simulink model "systolicArrayFinal"  (R2021a)
settings: Solver=VariableStepAuto  StartTime=0.0  StopTime=13  RelTol=1e-3
libraries: hdlBasic x120, xbsIndex_r4 x1
(part 1 of 2)
settings Model: Creator=caval  LastModifiedBy=kv25

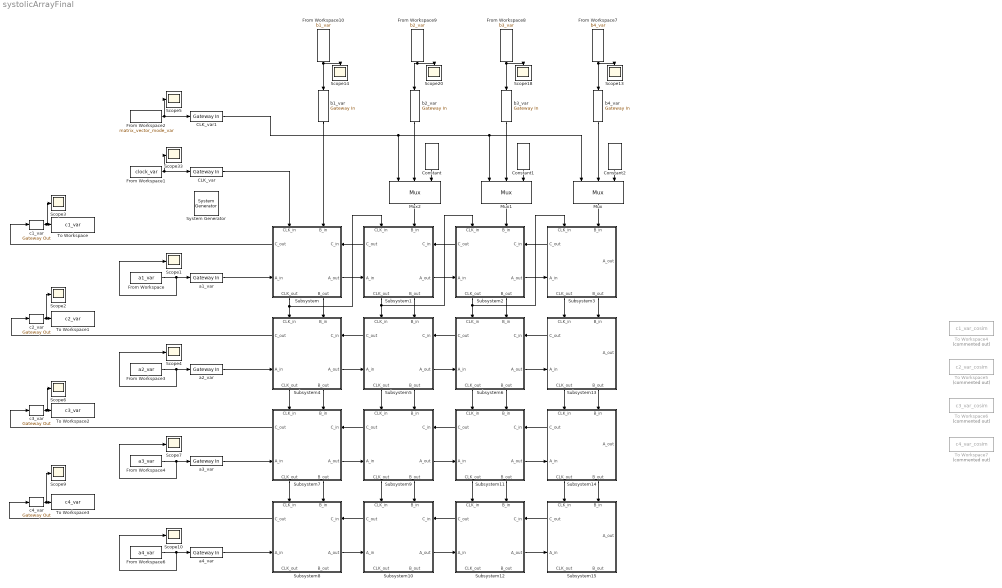
== system systolicArrayFinal ==
  " System Generator" : xbsIndex_r4/ System Generator  Tag=genX  xilinxfamily=zynq  part=xc7z020  speed=-1  package=clg484  synthesis_tool=Vivado  clock_wrapper=Clock Enables  directory=./netlist5  proj_type=Vivado  Synth_file=Vivado Synthesis Defaults  Impl_file=Vivado Implementation Defaults  testbench=off  simulink_period=1  sysclk_period=7  dcm_input_clock_period=10  incr_netlist=off  trim_vbits=Everywhere in SubSystem  dbl_ovrd=According to Block Masks  core_generation=According to Block Masks  run_coregen=off  deprecated_control=off  eval_field=0  block_type=sysgen
  CLK_var : hdlBasic/Gateway In  gui_display_data_type=Boolean  arith_type=Boolean  n_bits=16  bin_pt=0  preci_type=Single  exp_width=8  frac_width=24  rows=1  columns=1  quantization="Round  (unbiased: +/- Inf)"  overflow=Saturate  period=1  UseAsADC=off  ADCChannel='1'  interface=None  automatic_assignment=on  address_offset=hex2dec('00')  intf_name=''  intf_description=''  default_value=0  timing_constraint=None  locs_specified=off  LOCs={}  io_standard={}  inherit_from_input=off  hdl_port=on  XmcBlockStatus=1  maskContainerNames=group4  block_type=gatewayin  block_config=sysgen:gateway_in_config  block_width_w=590  block_height_w=620  block_width=640  block_height=850
  CLK_var1 : hdlBasic/Gateway In  gui_display_data_type=Boolean  arith_type=Boolean  n_bits=16  bin_pt=0  preci_type=Single  exp_width=8  frac_width=24  rows=1  columns=1  quantization="Round  (unbiased: +/- Inf)"  overflow=Saturate  period=1  UseAsADC=off  ADCChannel='1'  interface=None  automatic_assignment=on  address_offset=hex2dec('00')  intf_name=''  intf_description=''  default_value=0  timing_constraint=None  locs_specified=off  LOCs={}  io_standard={}  inherit_from_input=off  hdl_port=on  XmcBlockStatus=1  maskContainerNames=group4  block_type=gatewayin  block_config=sysgen:gateway_in_config  block_width_w=590  block_height_w=620  block_width=640  block_height=850
  Constant : hdlBasic/Constant  const=0  gui_display_data_type=Fixed-point  arith_type=Signed (2's comp)  n_bits=16  bin_pt=0  preci_type=Single  exp_width=8  frac_width=24  explicit_period=off  period=1  XmcBlockStatus=1  maskContainerNames=tabcontainer1  block_type=constant  block_config=sysgen:Constant_config
  Constant1 : hdlBasic/Constant  const=0  gui_display_data_type=Fixed-point  arith_type=Signed (2's comp)  n_bits=16  bin_pt=0  preci_type=Single  exp_width=8  frac_width=24  explicit_period=off  period=1  XmcBlockStatus=1  maskContainerNames=tabcontainer1  block_type=constant  block_config=sysgen:Constant_config
  Constant2 : hdlBasic/Constant  const=0  gui_display_data_type=Fixed-point  arith_type=Signed (2's comp)  n_bits=16  bin_pt=0  preci_type=Single  exp_width=8  frac_width=24  explicit_period=off  period=1  XmcBlockStatus=1  maskContainerNames=tabcontainer1  block_type=constant  block_config=sysgen:Constant_config
  From Workspace : FromWorkspace  VariableName=a1_var
  From Workspace1 : FromWorkspace  VariableName=clock_var
  From Workspace10 : FromWorkspace  VariableName=b1_var
  From Workspace2 : FromWorkspace  VariableName=matrix_vector_mode_var
  From Workspace3 : FromWorkspace  VariableName=a2_var
  From Workspace4 : FromWorkspace  VariableName=a3_var
  From Workspace6 : FromWorkspace  VariableName=a4_var
  From Workspace7 : FromWorkspace  VariableName=b4_var
  From Workspace8 : FromWorkspace  VariableName=b3_var
  From Workspace9 : FromWorkspace  VariableName=b2_var
  Mux : hdlBasic/Mux  inputs=2  en=off  latency=0  precision=Full  arith_type=Unsigned  n_bits=16  bin_pt=14  quantization=Truncate  overflow=Wrap  XmcBlockStatus=1  maskContainerNames=tabcontainer1  block_type=mux  block_config=sysgen:Mux_config
  Mux1 : hdlBasic/Mux  inputs=2  en=off  latency=0  precision=Full  arith_type=Unsigned  n_bits=16  bin_pt=14  quantization=Truncate  overflow=Wrap  XmcBlockStatus=1  maskContainerNames=tabcontainer1  block_type=mux  block_config=sysgen:Mux_config
  Mux2 : hdlBasic/Mux  inputs=2  en=off  latency=0  precision=Full  arith_type=Unsigned  n_bits=16  bin_pt=14  quantization=Truncate  overflow=Wrap  XmcBlockStatus=1  maskContainerNames=tabcontainer1  block_type=mux  block_config=sysgen:Mux_config
  Scope{1..7,9..10,13..14,18,20,33} (14 alike) : Scope
      Scope2 settings: Description=C14  AttributesFormatString=texttest
      Scope3 settings: Description=C14  AttributesFormatString=texttest
      Scope6 settings: Description=C14  AttributesFormatString=texttest
      Scope9 settings: Description=C14  AttributesFormatString=texttest
  Subsystem : Subsystem
      settings: PortSchema="{\"entries\":[{\"content\":{\"sides\":[{\"content\":{\"connectorIds\":[\"In1\",\"In2\"]},\"type\":\"ConnectorPlacement.EquallySpacedRectSide\",\"uuid\":\"d43d3dc0-f2a2-4485-9cc8-fdcdc63c7c64\"},{\"content\":{\"connectorIds\":[\"Out1\",\"Out2\"],\"side\":\"RIGHT\"},\"type\":\"ConnectorPlacement.EquallySpacedRectSide\",\"uuid\":\"56044226-4723-40c7-a478-8333213a0054\"},{\"content\":{\"connectorIds\":[\"Out4\",\"In3\"],\"side\":\"TOP\"},\"type\":\"ConnectorPlacement.EquallySpacedRectSide\",\"uuid\":\"fc372aae-6eb0-4644-b08a-28c78073ed8c\"},{\"content\":{\"connectorIds\":[\"In4\",\"Out3\"],\"side\":\"BOTTOM\"},\"type\":\"ConnectorPlacement.EquallySpacedRectSide\",\"uuid\":\"a99b4862-bd6b-40ce-bb78-73155b1cda06\"}]},\"type\":\"ConnectorPlacement.EquallySpacedConnector\",\"uuid\":\"00547539-55f6-42ab-bc8f-0525219f70ea\"}],\"packageUris\":[\"http://schema.mathworks.com/mf0/Connector/R2020b\"],\"version\":\"1.0\"}"
  Subsystem1 : Subsystem
      settings: PortSchema="{\"entries\":[{\"content\":{\"sides\":[{\"content\":{\"connectorIds\":[\"In1\",\"In2\"]},\"type\":\"ConnectorPlacement.EquallySpacedRectSide\",\"uuid\":\"d43d3dc0-f2a2-4485-9cc8-fdcdc63c7c64\"},{\"content\":{\"connectorIds\":[\"Out1\",\"Out2\"],\"side\":\"RIGHT\"},\"type\":\"ConnectorPlacement.EquallySpacedRectSide\",\"uuid\":\"56044226-4723-40c7-a478-8333213a0054\"},{\"content\":{\"connectorIds\":[\"Out4\",\"In3\"],\"side\":\"TOP\"},\"type\":\"ConnectorPlacement.EquallySpacedRectSide\",\"uuid\":\"fc372aae-6eb0-4644-b08a-28c78073ed8c\"},{\"content\":{\"connectorIds\":[\"In4\",\"Out3\"],\"side\":\"BOTTOM\"},\"type\":\"ConnectorPlacement.EquallySpacedRectSide\",\"uuid\":\"a99b4862-bd6b-40ce-bb78-73155b1cda06\"}]},\"type\":\"ConnectorPlacement.EquallySpacedConnector\",\"uuid\":\"00547539-55f6-42ab-bc8f-0525219f70ea\"}],\"packageUris\":[\"http://schema.mathworks.com/mf0/Connector/R2020b\"],\"version\":\"1.0\"}"
  Subsystem10 : Subsystem
      settings: PortSchema="{\"entries\":[{\"content\":{\"sides\":[{\"content\":{\"connectorIds\":[\"In1\",\"In2\"]},\"type\":\"ConnectorPlacement.EquallySpacedRectSide\",\"uuid\":\"d43d3dc0-f2a2-4485-9cc8-fdcdc63c7c64\"},{\"content\":{\"connectorIds\":[\"Out1\",\"Out2\"],\"side\":\"RIGHT\"},\"type\":\"ConnectorPlacement.EquallySpacedRectSide\",\"uuid\":\"56044226-4723-40c7-a478-8333213a0054\"},{\"content\":{\"connectorIds\":[\"Out4\",\"In3\"],\"side\":\"TOP\"},\"type\":\"ConnectorPlacement.EquallySpacedRectSide\",\"uuid\":\"fc372aae-6eb0-4644-b08a-28c78073ed8c\"},{\"content\":{\"connectorIds\":[\"In4\",\"Out3\"],\"side\":\"BOTTOM\"},\"type\":\"ConnectorPlacement.EquallySpacedRectSide\",\"uuid\":\"a99b4862-bd6b-40ce-bb78-73155b1cda06\"}]},\"type\":\"ConnectorPlacement.EquallySpacedConnector\",\"uuid\":\"00547539-55f6-42ab-bc8f-0525219f70ea\"}],\"packageUris\":[\"http://schema.mathworks.com/mf0/Connector/R2020b\"],\"version\":\"1.0\"}"
  Subsystem11 : Subsystem
      settings: PortSchema="{\"entries\":[{\"content\":{\"sides\":[{\"content\":{\"connectorIds\":[\"In1\",\"In2\"]},\"type\":\"ConnectorPlacement.EquallySpacedRectSide\",\"uuid\":\"d43d3dc0-f2a2-4485-9cc8-fdcdc63c7c64\"},{\"content\":{\"connectorIds\":[\"Out1\",\"Out2\"],\"side\":\"RIGHT\"},\"type\":\"ConnectorPlacement.EquallySpacedRectSide\",\"uuid\":\"56044226-4723-40c7-a478-8333213a0054\"},{\"content\":{\"connectorIds\":[\"Out4\",\"In3\"],\"side\":\"TOP\"},\"type\":\"ConnectorPlacement.EquallySpacedRectSide\",\"uuid\":\"fc372aae-6eb0-4644-b08a-28c78073ed8c\"},{\"content\":{\"connectorIds\":[\"In4\",\"Out3\"],\"side\":\"BOTTOM\"},\"type\":\"ConnectorPlacement.EquallySpacedRectSide\",\"uuid\":\"a99b4862-bd6b-40ce-bb78-73155b1cda06\"}]},\"type\":\"ConnectorPlacement.EquallySpacedConnector\",\"uuid\":\"00547539-55f6-42ab-bc8f-0525219f70ea\"}],\"packageUris\":[\"http://schema.mathworks.com/mf0/Connector/R2020b\"],\"version\":\"1.0\"}"
  Subsystem12 : Subsystem
      settings: PortSchema="{\"entries\":[{\"content\":{\"sides\":[{\"content\":{\"connectorIds\":[\"In1\",\"In2\"]},\"type\":\"ConnectorPlacement.EquallySpacedRectSide\",\"uuid\":\"d43d3dc0-f2a2-4485-9cc8-fdcdc63c7c64\"},{\"content\":{\"connectorIds\":[\"Out1\",\"Out2\"],\"side\":\"RIGHT\"},\"type\":\"ConnectorPlacement.EquallySpacedRectSide\",\"uuid\":\"56044226-4723-40c7-a478-8333213a0054\"},{\"content\":{\"connectorIds\":[\"Out4\",\"In3\"],\"side\":\"TOP\"},\"type\":\"ConnectorPlacement.EquallySpacedRectSide\",\"uuid\":\"fc372aae-6eb0-4644-b08a-28c78073ed8c\"},{\"content\":{\"connectorIds\":[\"In4\",\"Out3\"],\"side\":\"BOTTOM\"},\"type\":\"ConnectorPlacement.EquallySpacedRectSide\",\"uuid\":\"a99b4862-bd6b-40ce-bb78-73155b1cda06\"}]},\"type\":\"ConnectorPlacement.EquallySpacedConnector\",\"uuid\":\"00547539-55f6-42ab-bc8f-0525219f70ea\"}],\"packageUris\":[\"http://schema.mathworks.com/mf0/Connector/R2020b\"],\"version\":\"1.0\"}"
  Subsystem13 : Subsystem
      settings: PortSchema="{\"entries\":[{\"content\":{\"sides\":[{\"content\":{\"connectorIds\":[\"In1\",\"In2\"]},\"type\":\"ConnectorPlacement.EquallySpacedRectSide\",\"uuid\":\"d43d3dc0-f2a2-4485-9cc8-fdcdc63c7c64\"},{\"content\":{\"connectorIds\":[\"Out1\",\"Out2\"],\"side\":\"RIGHT\"},\"type\":\"ConnectorPlacement.EquallySpacedRectSide\",\"uuid\":\"56044226-4723-40c7-a478-8333213a0054\"},{\"content\":{\"connectorIds\":[\"Out4\",\"In3\"],\"side\":\"TOP\"},\"type\":\"ConnectorPlacement.EquallySpacedRectSide\",\"uuid\":\"fc372aae-6eb0-4644-b08a-28c78073ed8c\"},{\"content\":{\"connectorIds\":[\"Out3\"],\"side\":\"BOTTOM\"},\"type\":\"ConnectorPlacement.EquallySpacedRectSide\",\"uuid\":\"a99b4862-bd6b-40ce-bb78-73155b1cda06\"}]},\"type\":\"ConnectorPlacement.EquallySpacedConnector\",\"uuid\":\"00547539-55f6-42ab-bc8f-0525219f70ea\"}],\"packageUris\":[\"http://schema.mathworks.com/mf0/Connector/R2020b\"],\"version\":\"1.0\"}"
  Subsystem14 : Subsystem
      settings: PortSchema="{\"entries\":[{\"content\":{\"sides\":[{\"content\":{\"connectorIds\":[\"In1\",\"In2\"]},\"type\":\"ConnectorPlacement.EquallySpacedRectSide\",\"uuid\":\"d43d3dc0-f2a2-4485-9cc8-fdcdc63c7c64\"},{\"content\":{\"connectorIds\":[\"Out1\",\"Out2\"],\"side\":\"RIGHT\"},\"type\":\"ConnectorPlacement.EquallySpacedRectSide\",\"uuid\":\"56044226-4723-40c7-a478-8333213a0054\"},{\"content\":{\"connectorIds\":[\"Out4\",\"In3\"],\"side\":\"TOP\"},\"type\":\"ConnectorPlacement.EquallySpacedRectSide\",\"uuid\":\"fc372aae-6eb0-4644-b08a-28c78073ed8c\"},{\"content\":{\"connectorIds\":[\"Out3\"],\"side\":\"BOTTOM\"},\"type\":\"ConnectorPlacement.EquallySpacedRectSide\",\"uuid\":\"a99b4862-bd6b-40ce-bb78-73155b1cda06\"}]},\"type\":\"ConnectorPlacement.EquallySpacedConnector\",\"uuid\":\"00547539-55f6-42ab-bc8f-0525219f70ea\"}],\"packageUris\":[\"http://schema.mathworks.com/mf0/Connector/R2020b\"],\"version\":\"1.0\"}"
  Subsystem15 : Subsystem
      settings: PortSchema="{\"entries\":[{\"content\":{\"sides\":[{\"content\":{\"connectorIds\":[\"In1\",\"In2\"]},\"type\":\"ConnectorPlacement.EquallySpacedRectSide\",\"uuid\":\"d43d3dc0-f2a2-4485-9cc8-fdcdc63c7c64\"},{\"content\":{\"connectorIds\":[\"Out1\",\"Out2\"],\"side\":\"RIGHT\"},\"type\":\"ConnectorPlacement.EquallySpacedRectSide\",\"uuid\":\"56044226-4723-40c7-a478-8333213a0054\"},{\"content\":{\"connectorIds\":[\"Out4\",\"In3\"],\"side\":\"TOP\"},\"type\":\"ConnectorPlacement.EquallySpacedRectSide\",\"uuid\":\"fc372aae-6eb0-4644-b08a-28c78073ed8c\"},{\"content\":{\"connectorIds\":[\"Out3\"],\"side\":\"BOTTOM\"},\"type\":\"ConnectorPlacement.EquallySpacedRectSide\",\"uuid\":\"a99b4862-bd6b-40ce-bb78-73155b1cda06\"}]},\"type\":\"ConnectorPlacement.EquallySpacedConnector\",\"uuid\":\"00547539-55f6-42ab-bc8f-0525219f70ea\"}],\"packageUris\":[\"http://schema.mathworks.com/mf0/Connector/R2020b\"],\"version\":\"1.0\"}"
  Subsystem2 : Subsystem
      settings: PortSchema="{\"entries\":[{\"content\":{\"sides\":[{\"content\":{\"connectorIds\":[\"In1\",\"In2\"]},\"type\":\"ConnectorPlacement.EquallySpacedRectSide\",\"uuid\":\"d43d3dc0-f2a2-4485-9cc8-fdcdc63c7c64\"},{\"content\":{\"connectorIds\":[\"Out1\",\"Out2\"],\"side\":\"RIGHT\"},\"type\":\"ConnectorPlacement.EquallySpacedRectSide\",\"uuid\":\"56044226-4723-40c7-a478-8333213a0054\"},{\"content\":{\"connectorIds\":[\"Out4\",\"In3\"],\"side\":\"TOP\"},\"type\":\"ConnectorPlacement.EquallySpacedRectSide\",\"uuid\":\"fc372aae-6eb0-4644-b08a-28c78073ed8c\"},{\"content\":{\"connectorIds\":[\"In4\",\"Out3\"],\"side\":\"BOTTOM\"},\"type\":\"ConnectorPlacement.EquallySpacedRectSide\",\"uuid\":\"a99b4862-bd6b-40ce-bb78-73155b1cda06\"}]},\"type\":\"ConnectorPlacement.EquallySpacedConnector\",\"uuid\":\"00547539-55f6-42ab-bc8f-0525219f70ea\"}],\"packageUris\":[\"http://schema.mathworks.com/mf0/Connector/R2020b\"],\"version\":\"1.0\"}"
  Subsystem3 : Subsystem
      settings: PortSchema="{\"entries\":[{\"content\":{\"sides\":[{\"content\":{\"connectorIds\":[\"In1\",\"In2\"]},\"type\":\"ConnectorPlacement.EquallySpacedRectSide\",\"uuid\":\"d43d3dc0-f2a2-4485-9cc8-fdcdc63c7c64\"},{\"content\":{\"connectorIds\":[\"Out1\",\"Out2\"],\"side\":\"RIGHT\"},\"type\":\"ConnectorPlacement.EquallySpacedRectSide\",\"uuid\":\"56044226-4723-40c7-a478-8333213a0054\"},{\"content\":{\"connectorIds\":[\"Out4\",\"In3\"],\"side\":\"TOP\"},\"type\":\"ConnectorPlacement.EquallySpacedRectSide\",\"uuid\":\"fc372aae-6eb0-4644-b08a-28c78073ed8c\"},{\"content\":{\"connectorIds\":[\"Out3\"],\"side\":\"BOTTOM\"},\"type\":\"ConnectorPlacement.EquallySpacedRectSide\",\"uuid\":\"a99b4862-bd6b-40ce-bb78-73155b1cda06\"}]},\"type\":\"ConnectorPlacement.EquallySpacedConnector\",\"uuid\":\"00547539-55f6-42ab-bc8f-0525219f70ea\"}],\"packageUris\":[\"http://schema.mathworks.com/mf0/Connector/R2020b\"],\"version\":\"1.0\"}"
  Subsystem4 : Subsystem
      settings: PortSchema="{\"entries\":[{\"content\":{\"sides\":[{\"content\":{\"connectorIds\":[\"In1\",\"In2\"]},\"type\":\"ConnectorPlacement.EquallySpacedRectSide\",\"uuid\":\"d43d3dc0-f2a2-4485-9cc8-fdcdc63c7c64\"},{\"content\":{\"connectorIds\":[\"Out1\",\"Out2\"],\"side\":\"RIGHT\"},\"type\":\"ConnectorPlacement.EquallySpacedRectSide\",\"uuid\":\"56044226-4723-40c7-a478-8333213a0054\"},{\"content\":{\"connectorIds\":[\"Out4\",\"In3\"],\"side\":\"TOP\"},\"type\":\"ConnectorPlacement.EquallySpacedRectSide\",\"uuid\":\"fc372aae-6eb0-4644-b08a-28c78073ed8c\"},{\"content\":{\"connectorIds\":[\"In4\",\"Out3\"],\"side\":\"BOTTOM\"},\"type\":\"ConnectorPlacement.EquallySpacedRectSide\",\"uuid\":\"a99b4862-bd6b-40ce-bb78-73155b1cda06\"}]},\"type\":\"ConnectorPlacement.EquallySpacedConnector\",\"uuid\":\"00547539-55f6-42ab-bc8f-0525219f70ea\"}],\"packageUris\":[\"http://schema.mathworks.com/mf0/Connector/R2020b\"],\"version\":\"1.0\"}"
  Subsystem5 : Subsystem
      settings: PortSchema="{\"entries\":[{\"content\":{\"sides\":[{\"content\":{\"connectorIds\":[\"In1\",\"In2\"]},\"type\":\"ConnectorPlacement.EquallySpacedRectSide\",\"uuid\":\"d43d3dc0-f2a2-4485-9cc8-fdcdc63c7c64\"},{\"content\":{\"connectorIds\":[\"Out1\",\"Out2\"],\"side\":\"RIGHT\"},\"type\":\"ConnectorPlacement.EquallySpacedRectSide\",\"uuid\":\"56044226-4723-40c7-a478-8333213a0054\"},{\"content\":{\"connectorIds\":[\"Out4\",\"In3\"],\"side\":\"TOP\"},\"type\":\"ConnectorPlacement.EquallySpacedRectSide\",\"uuid\":\"fc372aae-6eb0-4644-b08a-28c78073ed8c\"},{\"content\":{\"connectorIds\":[\"In4\",\"Out3\"],\"side\":\"BOTTOM\"},\"type\":\"ConnectorPlacement.EquallySpacedRectSide\",\"uuid\":\"a99b4862-bd6b-40ce-bb78-73155b1cda06\"}]},\"type\":\"ConnectorPlacement.EquallySpacedConnector\",\"uuid\":\"00547539-55f6-42ab-bc8f-0525219f70ea\"}],\"packageUris\":[\"http://schema.mathworks.com/mf0/Connector/R2020b\"],\"version\":\"1.0\"}"
  Subsystem6 : Subsystem
      settings: PortSchema="{\"entries\":[{\"content\":{\"sides\":[{\"content\":{\"connectorIds\":[\"In1\",\"In2\"]},\"type\":\"ConnectorPlacement.EquallySpacedRectSide\",\"uuid\":\"d43d3dc0-f2a2-4485-9cc8-fdcdc63c7c64\"},{\"content\":{\"connectorIds\":[\"Out1\",\"Out2\"],\"side\":\"RIGHT\"},\"type\":\"ConnectorPlacement.EquallySpacedRectSide\",\"uuid\":\"56044226-4723-40c7-a478-8333213a0054\"},{\"content\":{\"connectorIds\":[\"Out4\",\"In3\"],\"side\":\"TOP\"},\"type\":\"ConnectorPlacement.EquallySpacedRectSide\",\"uuid\":\"fc372aae-6eb0-4644-b08a-28c78073ed8c\"},{\"content\":{\"connectorIds\":[\"In4\",\"Out3\"],\"side\":\"BOTTOM\"},\"type\":\"ConnectorPlacement.EquallySpacedRectSide\",\"uuid\":\"a99b4862-bd6b-40ce-bb78-73155b1cda06\"}]},\"type\":\"ConnectorPlacement.EquallySpacedConnector\",\"uuid\":\"00547539-55f6-42ab-bc8f-0525219f70ea\"}],\"packageUris\":[\"http://schema.mathworks.com/mf0/Connector/R2020b\"],\"version\":\"1.0\"}"
  Subsystem7 : Subsystem
      settings: PortSchema="{\"entries\":[{\"content\":{\"sides\":[{\"content\":{\"connectorIds\":[\"In1\",\"In2\"]},\"type\":\"ConnectorPlacement.EquallySpacedRectSide\",\"uuid\":\"d43d3dc0-f2a2-4485-9cc8-fdcdc63c7c64\"},{\"content\":{\"connectorIds\":[\"Out1\",\"Out2\"],\"side\":\"RIGHT\"},\"type\":\"ConnectorPlacement.EquallySpacedRectSide\",\"uuid\":\"56044226-4723-40c7-a478-8333213a0054\"},{\"content\":{\"connectorIds\":[\"Out4\",\"In3\"],\"side\":\"TOP\"},\"type\":\"ConnectorPlacement.EquallySpacedRectSide\",\"uuid\":\"fc372aae-6eb0-4644-b08a-28c78073ed8c\"},{\"content\":{\"connectorIds\":[\"In4\",\"Out3\"],\"side\":\"BOTTOM\"},\"type\":\"ConnectorPlacement.EquallySpacedRectSide\",\"uuid\":\"a99b4862-bd6b-40ce-bb78-73155b1cda06\"}]},\"type\":\"ConnectorPlacement.EquallySpacedConnector\",\"uuid\":\"00547539-55f6-42ab-bc8f-0525219f70ea\"}],\"packageUris\":[\"http://schema.mathworks.com/mf0/Connector/R2020b\"],\"version\":\"1.0\"}"
  Subsystem8 : Subsystem
      settings: PortSchema="{\"entries\":[{\"content\":{\"sides\":[{\"content\":{\"connectorIds\":[\"In1\",\"In2\"]},\"type\":\"ConnectorPlacement.EquallySpacedRectSide\",\"uuid\":\"d43d3dc0-f2a2-4485-9cc8-fdcdc63c7c64\"},{\"content\":{\"connectorIds\":[\"Out1\",\"Out2\"],\"side\":\"RIGHT\"},\"type\":\"ConnectorPlacement.EquallySpacedRectSide\",\"uuid\":\"56044226-4723-40c7-a478-8333213a0054\"},{\"content\":{\"connectorIds\":[\"Out4\",\"In3\"],\"side\":\"TOP\"},\"type\":\"ConnectorPlacement.EquallySpacedRectSide\",\"uuid\":\"fc372aae-6eb0-4644-b08a-28c78073ed8c\"},{\"content\":{\"connectorIds\":[\"In4\",\"Out3\"],\"side\":\"BOTTOM\"},\"type\":\"ConnectorPlacement.EquallySpacedRectSide\",\"uuid\":\"a99b4862-bd6b-40ce-bb78-73155b1cda06\"}]},\"type\":\"ConnectorPlacement.EquallySpacedConnector\",\"uuid\":\"00547539-55f6-42ab-bc8f-0525219f70ea\"}],\"packageUris\":[\"http://schema.mathworks.com/mf0/Connector/R2020b\"],\"version\":\"1.0\"}"
  Subsystem9 : Subsystem
      settings: PortSchema="{\"entries\":[{\"content\":{\"sides\":[{\"content\":{\"connectorIds\":[\"In1\",\"In2\"]},\"type\":\"ConnectorPlacement.EquallySpacedRectSide\",\"uuid\":\"d43d3dc0-f2a2-4485-9cc8-fdcdc63c7c64\"},{\"content\":{\"connectorIds\":[\"Out1\",\"Out2\"],\"side\":\"RIGHT\"},\"type\":\"ConnectorPlacement.EquallySpacedRectSide\",\"uuid\":\"56044226-4723-40c7-a478-8333213a0054\"},{\"content\":{\"connectorIds\":[\"Out4\",\"In3\"],\"side\":\"TOP\"},\"type\":\"ConnectorPlacement.EquallySpacedRectSide\",\"uuid\":\"fc372aae-6eb0-4644-b08a-28c78073ed8c\"},{\"content\":{\"connectorIds\":[\"In4\",\"Out3\"],\"side\":\"BOTTOM\"},\"type\":\"ConnectorPlacement.EquallySpacedRectSide\",\"uuid\":\"a99b4862-bd6b-40ce-bb78-73155b1cda06\"}]},\"type\":\"ConnectorPlacement.EquallySpacedConnector\",\"uuid\":\"00547539-55f6-42ab-bc8f-0525219f70ea\"}],\"packageUris\":[\"http://schema.mathworks.com/mf0/Connector/R2020b\"],\"version\":\"1.0\"}"
  To Workspace : ToWorkspace  VariableName=c1_var  SaveFormat=Timeseries  SampleTime=-1
  To Workspace1 : ToWorkspace  VariableName=c2_var  SaveFormat=Timeseries  SampleTime=-1
  To Workspace2 : ToWorkspace  VariableName=c3_var  SaveFormat=Timeseries  SampleTime=-1
  To Workspace3 : ToWorkspace  VariableName=c4_var  SaveFormat=Timeseries  SampleTime=-1
  To Workspace4 : ToWorkspace  Commented=on  VariableName=c1_var_cosim  SaveFormat=Timeseries  SampleTime=-1
  To Workspace5 : ToWorkspace  Commented=on  VariableName=c2_var_cosim  SaveFormat=Timeseries  SampleTime=-1
  To Workspace6 : ToWorkspace  Commented=on  VariableName=c3_var_cosim  SaveFormat=Timeseries  SampleTime=-1
  To Workspace7 : ToWorkspace  Commented=on  VariableName=c4_var_cosim  SaveFormat=Timeseries  SampleTime=-1
  a1_var : hdlBasic/Gateway In  gui_display_data_type=Fixed-point  arith_type=Signed (2's comp)  n_bits=16  bin_pt=0  preci_type=Single  exp_width=8  frac_width=24  rows=1  columns=1  quantization="Round  (unbiased: +/- Inf)"  overflow=Saturate  period=1  UseAsADC=off  ADCChannel='1'  interface=None  automatic_assignment=on  address_offset=hex2dec('00')  intf_name=''  intf_description=''  default_value=0  timing_constraint=None  locs_specified=off  LOCs={}  io_standard={}  inherit_from_input=off  hdl_port=on  XmcBlockStatus=1  maskContainerNames=group4  block_type=gatewayin  block_config=sysgen:gateway_in_config  block_width_w=590  block_height_w=620  block_width=640  block_height=850
  a2_var : hdlBasic/Gateway In  gui_display_data_type=Fixed-point  arith_type=Signed (2's comp)  n_bits=16  bin_pt=0  preci_type=Single  exp_width=8  frac_width=24  rows=1  columns=1  quantization="Round  (unbiased: +/- Inf)"  overflow=Saturate  period=1  UseAsADC=off  ADCChannel='1'  interface=None  automatic_assignment=on  address_offset=hex2dec('00')  intf_name=''  intf_description=''  default_value=0  timing_constraint=None  locs_specified=off  LOCs={}  io_standard={}  inherit_from_input=off  hdl_port=on  XmcBlockStatus=1  maskContainerNames=group4  block_type=gatewayin  block_config=sysgen:gateway_in_config  block_width_w=590  block_height_w=620  block_width=640  block_height=850
  a3_var : hdlBasic/Gateway In  gui_display_data_type=Fixed-point  arith_type=Signed (2's comp)  n_bits=16  bin_pt=0  preci_type=Single  exp_width=8  frac_width=24  rows=1  columns=1  quantization="Round  (unbiased: +/- Inf)"  overflow=Saturate  period=1  UseAsADC=off  ADCChannel='1'  interface=None  automatic_assignment=on  address_offset=hex2dec('00')  intf_name=''  intf_description=''  default_value=0  timing_constraint=None  locs_specified=off  LOCs={}  io_standard={}  inherit_from_input=off  hdl_port=on  XmcBlockStatus=1  maskContainerNames=group4  block_type=gatewayin  block_config=sysgen:gateway_in_config  block_width_w=590  block_height_w=620  block_width=640  block_height=850
  a4_var : hdlBasic/Gateway In  gui_display_data_type=Fixed-point  arith_type=Signed (2's comp)  n_bits=16  bin_pt=0  preci_type=Single  exp_width=8  frac_width=24  rows=1  columns=1  quantization="Round  (unbiased: +/- Inf)"  overflow=Saturate  period=1  UseAsADC=off  ADCChannel='1'  interface=None  automatic_assignment=on  address_offset=hex2dec('00')  intf_name=''  intf_description=''  default_value=0  timing_constraint=None  locs_specified=off  LOCs={}  io_standard={}  inherit_from_input=off  hdl_port=on  XmcBlockStatus=1  maskContainerNames=group4  block_type=gatewayin  block_config=sysgen:gateway_in_config  block_width_w=590  block_height_w=620  block_width=640  block_height=850
  b1_var : hdlBasic/Gateway In  gui_display_data_type=Fixed-point  arith_type=Signed (2's comp)  n_bits=16  bin_pt=0  preci_type=Single  exp_width=8  frac_width=24  rows=1  columns=1  quantization="Round  (unbiased: +/- Inf)"  overflow=Saturate  period=1  UseAsADC=off  ADCChannel='1'  interface=None  automatic_assignment=on  address_offset=hex2dec('00')  intf_name=''  intf_description=''  default_value=0  timing_constraint=None  locs_specified=off  LOCs={}  io_standard={}  inherit_from_input=off  hdl_port=on  XmcBlockStatus=1  maskContainerNames=group4  block_type=gatewayin  block_config=sysgen:gateway_in_config  block_width_w=590  block_height_w=620  block_width=640  block_height=850
  b2_var : hdlBasic/Gateway In  gui_display_data_type=Fixed-point  arith_type=Signed (2's comp)  n_bits=16  bin_pt=0  preci_type=Single  exp_width=8  frac_width=24  rows=1  columns=1  quantization="Round  (unbiased: +/- Inf)"  overflow=Saturate  period=1  UseAsADC=off  ADCChannel='1'  interface=None  automatic_assignment=on  address_offset=hex2dec('00')  intf_name=''  intf_description=''  default_value=0  timing_constraint=None  locs_specified=off  LOCs={}  io_standard={}  inherit_from_input=off  hdl_port=on  XmcBlockStatus=1  maskContainerNames=group4  block_type=gatewayin  block_config=sysgen:gateway_in_config  block_width_w=590  block_height_w=620  block_width=640  block_height=850
  b3_var : hdlBasic/Gateway In  gui_display_data_type=Fixed-point  arith_type=Signed (2's comp)  n_bits=16  bin_pt=0  preci_type=Single  exp_width=8  frac_width=24  rows=1  columns=1  quantization="Round  (unbiased: +/- Inf)"  overflow=Saturate  period=1  UseAsADC=off  ADCChannel='1'  interface=None  automatic_assignment=on  address_offset=hex2dec('00')  intf_name=''  intf_description=''  default_value=0  timing_constraint=None  locs_specified=off  LOCs={}  io_standard={}  inherit_from_input=off  hdl_port=on  XmcBlockStatus=1  maskContainerNames=group4  block_type=gatewayin  block_config=sysgen:gateway_in_config  block_width_w=590  block_height_w=620  block_width=640  block_height=850
  b4_var : hdlBasic/Gateway In  gui_display_data_type=Fixed-point  arith_type=Signed (2's comp)  n_bits=16  bin_pt=0  preci_type=Single  exp_width=8  frac_width=24  rows=1  columns=1  quantization="Round  (unbiased: +/- Inf)"  overflow=Saturate  period=1  UseAsADC=off  ADCChannel='1'  interface=None  automatic_assignment=on  address_offset=hex2dec('00')  intf_name=''  intf_description=''  default_value=0  timing_constraint=None  locs_specified=off  LOCs={}  io_standard={}  inherit_from_input=off  hdl_port=on  XmcBlockStatus=1  maskContainerNames=group4  block_type=gatewayin  block_config=sysgen:gateway_in_config  block_width_w=590  block_height_w=620  block_width=640  block_height=850
  c1_var : hdlBasic/Gateway Out  inherit_from_input=off  hdl_port=on  rows=1  columns=1  UseAsDAC=off  DACChannel='1'  interface=None  automatic_assignment=on  address_offset=hex2dec('00')  intf_name=''  intf_description=''  timing_constraint=None  locs_specified=off  LOCs={}  io_standard={}  XmcBlockStatus=1  maskContainerNames=group4  block_type=gatewayout  block_config=sysgen:gateway_out_config  block_width_w=590  block_height_w=620  block_width=620  block_height=750
  c2_var : hdlBasic/Gateway Out  inherit_from_input=off  hdl_port=on  rows=1  columns=1  UseAsDAC=off  DACChannel='1'  interface=None  automatic_assignment=on  address_offset=hex2dec('00')  intf_name=''  intf_description=''  timing_constraint=None  locs_specified=off  LOCs={}  io_standard={}  XmcBlockStatus=1  maskContainerNames=group4  block_type=gatewayout  block_config=sysgen:gateway_out_config  block_width_w=590  block_height_w=620  block_width=620  block_height=750
  c3_var : hdlBasic/Gateway Out  inherit_from_input=off  hdl_port=on  rows=1  columns=1  UseAsDAC=off  DACChannel='1'  interface=None  automatic_assignment=on  address_offset=hex2dec('00')  intf_name=''  intf_description=''  timing_constraint=None  locs_specified=off  LOCs={}  io_standard={}  XmcBlockStatus=1  maskContainerNames=group4  block_type=gatewayout  block_config=sysgen:gateway_out_config  block_width_w=590  block_height_w=620  block_width=620  block_height=750
  c4_var : hdlBasic/Gateway Out  inherit_from_input=off  hdl_port=on  rows=1  columns=1  UseAsDAC=off  DACChannel='1'  interface=None  automatic_assignment=on  address_offset=hex2dec('00')  intf_name=''  intf_description=''  timing_constraint=None  locs_specified=off  LOCs={}  io_standard={}  XmcBlockStatus=1  maskContainerNames=group4  block_type=gatewayout  block_config=sysgen:gateway_out_config  block_width_w=590  block_height_w=620  block_width=620  block_height=750
  wires:
  From Workspace/1 -> Scope1/1, a1_var/1
  From Workspace3/1 -> Scope4/1, a2_var/1
  From Workspace6/1 -> Scope10/1, a4_var/1
  From Workspace4/1 -> Scope7/1, a3_var/1
  From Workspace8/1 -> Scope18/1, b3_var/1
  From Workspace10/1 -> Scope14/1, b1_var/1
  From Workspace9/1 -> Scope20/1, b2_var/1
  From Workspace7/1 -> Scope13/1, b4_var/1
  a1_var/1 -> Subsystem/3(A_in)
  Subsystem/3(A_out) -> Subsystem1/3(A_in)
  Subsystem1/3(A_out) -> Subsystem2/3(A_in)
  Subsystem2/3(A_out) -> Subsystem3/3(A_in)
  Subsystem4/3(A_out) -> Subsystem5/3(A_in)
  Subsystem5/3(A_out) -> Subsystem6/3(A_in)
  Subsystem6/3(A_out) -> Subsystem13/3(A_in)
  Subsystem7/3(A_out) -> Subsystem9/3(A_in)
  Subsystem9/3(A_out) -> Subsystem11/3(A_in)
  Subsystem11/3(A_out) -> Subsystem14/3(A_in)
  Subsystem8/3(A_out) -> Subsystem10/3(A_in)
  Subsystem10/3(A_out) -> Subsystem12/3(A_in)
  Subsystem12/3(A_out) -> Subsystem15/3(A_in)
  a2_var/1 -> Subsystem4/3(A_in)
  a3_var/1 -> Subsystem7/3(A_in)
  a4_var/1 -> Subsystem8/3(A_in)
  b1_var/1 -> Subsystem/2(B_in)
  CLK_var/1 -> Subsystem/1(CLK_in)
  Subsystem4/1(CLK_out) -> Subsystem7/1(CLK_in)
  Subsystem7/1(CLK_out) -> Subsystem8/1(CLK_in)
  Subsystem5/1(CLK_out) -> Subsystem9/1(CLK_in)
  Subsystem9/1(CLK_out) -> Subsystem10/1(CLK_in)
  Subsystem6/1(CLK_out) -> Subsystem11/1(CLK_in)
  Subsystem11/1(CLK_out) -> Subsystem12/1(CLK_in)
  Subsystem14/1(CLK_out) -> Subsystem15/1(CLK_in)
  Subsystem3/1(CLK_out) -> Subsystem13/1(CLK_in)
  Subsystem3/4(C_out) -> Subsystem2/4(C_in)
  Subsystem2/4(C_out) -> Subsystem1/4(C_in)
  Subsystem1/4(C_out) -> Subsystem/4(C_in)
  Subsystem5/4(C_out) -> Subsystem4/4(C_in)
  Subsystem6/4(C_out) -> Subsystem5/4(C_in)
  Subsystem13/4(C_out) -> Subsystem6/4(C_in)
  Subsystem9/4(C_out) -> Subsystem7/4(C_in)
  Subsystem11/4(C_out) -> Subsystem9/4(C_in)
  Subsystem14/4(C_out) -> Subsystem11/4(C_in)
  Subsystem15/4(C_out) -> Subsystem12/4(C_in)
  Subsystem12/4(C_out) -> Subsystem10/4(C_in)
  Subsystem10/4(C_out) -> Subsystem8/4(C_in)
  Subsystem8/4(C_out) -> c4_var/1
  c4_var/1 -> Scope9/1, To Workspace3/1
  c3_var/1 -> Scope6/1, To Workspace2/1
  c1_var/1 -> Scope3/1, To Workspace/1
  c2_var/1 -> Scope2/1, To Workspace1/1
  Subsystem7/4(C_out) -> c3_var/1
  Subsystem4/4(C_out) -> c2_var/1
  Subsystem/4(C_out) -> c1_var/1
  Subsystem1/2(B_out) -> Subsystem5/2(B_in)
  Subsystem5/2(B_out) -> Subsystem9/2(B_in)
  Subsystem9/2(B_out) -> Subsystem10/2(B_in)
  Subsystem11/2(B_out) -> Subsystem12/2(B_in)
  Subsystem14/2(B_out) -> Subsystem15/2(B_in)
  Subsystem6/2(B_out) -> Subsystem11/2(B_in)
  Subsystem3/2(B_out) -> Subsystem13/2(B_in)
  Subsystem2/2(B_out) -> Subsystem6/2(B_in)
  Subsystem/2(B_out) -> Subsystem4/2(B_in)
  Subsystem4/2(B_out) -> Subsystem7/2(B_in)
  Subsystem7/2(B_out) -> Subsystem8/2(B_in)
  Subsystem13/1(CLK_out) -> Subsystem14/1(CLK_in)
  Subsystem13/2(B_out) -> Subsystem14/2(B_in)
  Subsystem2/1(CLK_out) -> Subsystem3/1(CLK_in), Subsystem6/1(CLK_in)
  Subsystem1/1(CLK_out) -> Subsystem2/1(CLK_in), Subsystem5/1(CLK_in)
  Subsystem/1(CLK_out) -> Subsystem1/1(CLK_in), Subsystem4/1(CLK_in)
  From Workspace1/1 -> Scope33/1, CLK_var/1
  From Workspace2/1 -> Scope5/1, CLK_var1/1
  Mux2/1 -> Subsystem1/2(B_in)
  Mux1/1 -> Subsystem2/2(B_in)
  Mux/1 -> Subsystem3/2(B_in)
  Constant/1 -> Mux2/3
  Constant2/1 -> Mux/3
  Constant1/1 -> Mux1/3
  b2_var/1 -> Mux2/2
  b3_var/1 -> Mux1/2
  b4_var/1 -> Mux/2
  CLK_var1/1 -> Mux2/1, Mux/1, Mux1/1
  ? -> To Workspace4/1
  ? -> To Workspace5/1
  ? -> To Workspace6/1
  ? -> To Workspace7/1

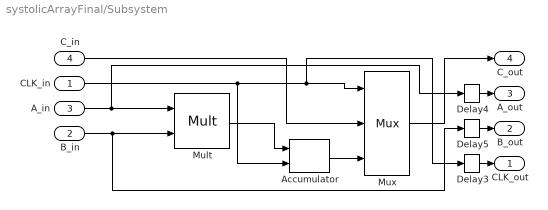
== system systolicArrayFinal/Subsystem ==
  CLK_in : Inport
  B_in : Inport  Port=2
  A_in : Inport  Port=3
  C_in : Inport  Port=4
  Accumulator : hdlBasic/Accumulator  operation=Add  n_bits=8  overflow=Wrap  scale=1  rst=on  hasbypass=off  en=off  latency=1  msb_inp=100  msb=100  lsb=-100  use_behavioral_HDL=on  implementation=Fabric  XmcBlockStatus=1  maskContainerNames=group3  block_type=accum  block_config=sysgen:Accum_config
  Delay3 : hdlBasic/Delay  rst=off  en=off  latency=1  reg_retiming=off  XmcBlockStatus=1  maskContainerNames=group1  block_type=delay  block_config=sysgen:Delay_config
  Delay4 : hdlBasic/Delay  rst=off  en=off  latency=1  reg_retiming=off  XmcBlockStatus=1  maskContainerNames=group1  block_type=delay  block_config=sysgen:Delay_config
  Delay5 : hdlBasic/Delay  rst=off  en=off  latency=1  reg_retiming=off  XmcBlockStatus=1  maskContainerNames=group1  block_type=delay  block_config=sysgen:Delay_config
  Mult : hdlBasic/Mult  precision=Full  arith_type="Signed  (2's comp)"  n_bits=16  bin_pt=14  quantization=Truncate  overflow=Wrap  en=off  latency=0  use_behavioral_HDL=off  opt=Speed  use_embedded=on  optimum_pipeline=off  pipeline=on  use_rpm=on  placement_style=Triangular  XmcBlockStatus=1  maskContainerNames=group1  block_type=mult  block_config=sysgen:Mult_config
  Mux : hdlBasic/Mux  inputs=2  en=off  latency=0  precision=Full  arith_type=Unsigned  n_bits=16  bin_pt=14  quantization=Truncate  overflow=Wrap  XmcBlockStatus=1  maskContainerNames=tabcontainer1  block_type=mux  block_config=sysgen:Mux_config
  CLK_out : Outport
  B_out : Outport  Port=2
  A_out : Outport  Port=3
  C_out : Outport  Port=4
  wires:
  Accumulator/1 -> Mux/3
  Mult/1 -> Accumulator/1
  Mux/1 -> C_out/1
  CLK_in/1 -> Accumulator/2, Delay3/1, Mux/1
  C_in/1 -> Mux/2
  A_in/1 -> Delay4/1, Mult/1
  B_in/1 -> Delay5/1, Mult/2
  Delay3/1 -> CLK_out/1
  Delay4/1 -> A_out/1
  Delay5/1 -> B_out/1

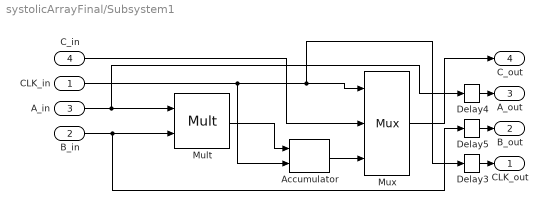
== system systolicArrayFinal/Subsystem1 ==
  CLK_in : Inport
  B_in : Inport  Port=2
  A_in : Inport  Port=3
  C_in : Inport  Port=4
  Accumulator : hdlBasic/Accumulator  operation=Add  n_bits=8  overflow=Wrap  scale=1  rst=on  hasbypass=off  en=off  latency=1  msb_inp=100  msb=100  lsb=-100  use_behavioral_HDL=on  implementation=Fabric  XmcBlockStatus=1  maskContainerNames=group3  block_type=accum  block_config=sysgen:Accum_config
  Delay3 : hdlBasic/Delay  rst=off  en=off  latency=1  reg_retiming=off  XmcBlockStatus=1  maskContainerNames=group1  block_type=delay  block_config=sysgen:Delay_config
  Delay4 : hdlBasic/Delay  rst=off  en=off  latency=1  reg_retiming=off  XmcBlockStatus=1  maskContainerNames=group1  block_type=delay  block_config=sysgen:Delay_config
  Delay5 : hdlBasic/Delay  rst=off  en=off  latency=1  reg_retiming=off  XmcBlockStatus=1  maskContainerNames=group1  block_type=delay  block_config=sysgen:Delay_config
  Mult : hdlBasic/Mult  precision=Full  arith_type="Signed  (2's comp)"  n_bits=16  bin_pt=14  quantization=Truncate  overflow=Wrap  en=off  latency=0  use_behavioral_HDL=off  opt=Speed  use_embedded=on  optimum_pipeline=off  pipeline=on  use_rpm=on  placement_style=Triangular  XmcBlockStatus=1  maskContainerNames=group1  block_type=mult  block_config=sysgen:Mult_config
  Mux : hdlBasic/Mux  inputs=2  en=off  latency=0  precision=Full  arith_type=Unsigned  n_bits=16  bin_pt=14  quantization=Truncate  overflow=Wrap  XmcBlockStatus=1  maskContainerNames=tabcontainer1  block_type=mux  block_config=sysgen:Mux_config
  CLK_out : Outport
  B_out : Outport  Port=2
  A_out : Outport  Port=3
  C_out : Outport  Port=4
  wires:
  Accumulator/1 -> Mux/3
  Mult/1 -> Accumulator/1
  Mux/1 -> C_out/1
  CLK_in/1 -> Accumulator/2, Delay3/1, Mux/1
  C_in/1 -> Mux/2
  A_in/1 -> Delay4/1, Mult/1
  B_in/1 -> Delay5/1, Mult/2
  Delay3/1 -> CLK_out/1
  Delay4/1 -> A_out/1
  Delay5/1 -> B_out/1

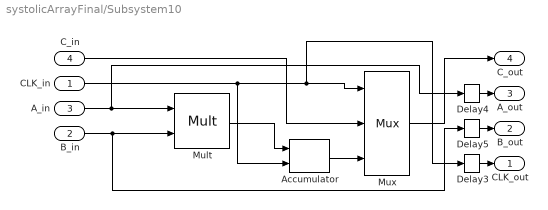
== system systolicArrayFinal/Subsystem10 ==
  CLK_in : Inport
  B_in : Inport  Port=2
  A_in : Inport  Port=3
  C_in : Inport  Port=4
  Accumulator : hdlBasic/Accumulator  operation=Add  n_bits=8  overflow=Wrap  scale=1  rst=on  hasbypass=off  en=off  latency=1  msb_inp=100  msb=100  lsb=-100  use_behavioral_HDL=on  implementation=Fabric  XmcBlockStatus=1  maskContainerNames=group3  block_type=accum  block_config=sysgen:Accum_config
  Delay3 : hdlBasic/Delay  rst=off  en=off  latency=1  reg_retiming=off  XmcBlockStatus=1  maskContainerNames=group1  block_type=delay  block_config=sysgen:Delay_config
  Delay4 : hdlBasic/Delay  rst=off  en=off  latency=1  reg_retiming=off  XmcBlockStatus=1  maskContainerNames=group1  block_type=delay  block_config=sysgen:Delay_config
  Delay5 : hdlBasic/Delay  rst=off  en=off  latency=1  reg_retiming=off  XmcBlockStatus=1  maskContainerNames=group1  block_type=delay  block_config=sysgen:Delay_config
  Mult : hdlBasic/Mult  precision=Full  arith_type="Signed  (2's comp)"  n_bits=16  bin_pt=14  quantization=Truncate  overflow=Wrap  en=off  latency=0  use_behavioral_HDL=off  opt=Speed  use_embedded=on  optimum_pipeline=off  pipeline=on  use_rpm=on  placement_style=Triangular  XmcBlockStatus=1  maskContainerNames=group1  block_type=mult  block_config=sysgen:Mult_config
  Mux : hdlBasic/Mux  inputs=2  en=off  latency=0  precision=Full  arith_type=Unsigned  n_bits=16  bin_pt=14  quantization=Truncate  overflow=Wrap  XmcBlockStatus=1  maskContainerNames=tabcontainer1  block_type=mux  block_config=sysgen:Mux_config
  CLK_out : Outport
  B_out : Outport  Port=2
  A_out : Outport  Port=3
  C_out : Outport  Port=4
  wires:
  Accumulator/1 -> Mux/3
  Mult/1 -> Accumulator/1
  Mux/1 -> C_out/1
  CLK_in/1 -> Accumulator/2, Delay3/1, Mux/1
  C_in/1 -> Mux/2
  A_in/1 -> Delay4/1, Mult/1
  B_in/1 -> Delay5/1, Mult/2
  Delay3/1 -> CLK_out/1
  Delay4/1 -> A_out/1
  Delay5/1 -> B_out/1

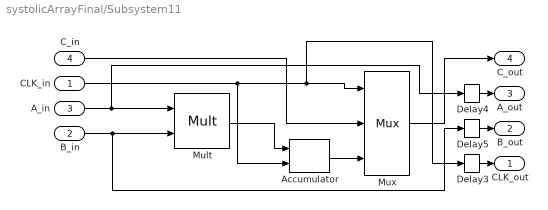
== system systolicArrayFinal/Subsystem11 ==
  CLK_in : Inport
  B_in : Inport  Port=2
  A_in : Inport  Port=3
  C_in : Inport  Port=4
  Accumulator : hdlBasic/Accumulator  operation=Add  n_bits=8  overflow=Wrap  scale=1  rst=on  hasbypass=off  en=off  latency=1  msb_inp=100  msb=100  lsb=-100  use_behavioral_HDL=on  implementation=Fabric  XmcBlockStatus=1  maskContainerNames=group3  block_type=accum  block_config=sysgen:Accum_config
  Delay3 : hdlBasic/Delay  rst=off  en=off  latency=1  reg_retiming=off  XmcBlockStatus=1  maskContainerNames=group1  block_type=delay  block_config=sysgen:Delay_config
  Delay4 : hdlBasic/Delay  rst=off  en=off  latency=1  reg_retiming=off  XmcBlockStatus=1  maskContainerNames=group1  block_type=delay  block_config=sysgen:Delay_config
  Delay5 : hdlBasic/Delay  rst=off  en=off  latency=1  reg_retiming=off  XmcBlockStatus=1  maskContainerNames=group1  block_type=delay  block_config=sysgen:Delay_config
  Mult : hdlBasic/Mult  precision=Full  arith_type="Signed  (2's comp)"  n_bits=16  bin_pt=14  quantization=Truncate  overflow=Wrap  en=off  latency=0  use_behavioral_HDL=off  opt=Speed  use_embedded=on  optimum_pipeline=off  pipeline=on  use_rpm=on  placement_style=Triangular  XmcBlockStatus=1  maskContainerNames=group1  block_type=mult  block_config=sysgen:Mult_config
  Mux : hdlBasic/Mux  inputs=2  en=off  latency=0  precision=Full  arith_type=Unsigned  n_bits=16  bin_pt=14  quantization=Truncate  overflow=Wrap  XmcBlockStatus=1  maskContainerNames=tabcontainer1  block_type=mux  block_config=sysgen:Mux_config
  CLK_out : Outport
  B_out : Outport  Port=2
  A_out : Outport  Port=3
  C_out : Outport  Port=4
  wires:
  Accumulator/1 -> Mux/3
  Mult/1 -> Accumulator/1
  Mux/1 -> C_out/1
  CLK_in/1 -> Accumulator/2, Delay3/1, Mux/1
  C_in/1 -> Mux/2
  A_in/1 -> Delay4/1, Mult/1
  B_in/1 -> Delay5/1, Mult/2
  Delay3/1 -> CLK_out/1
  Delay4/1 -> A_out/1
  Delay5/1 -> B_out/1

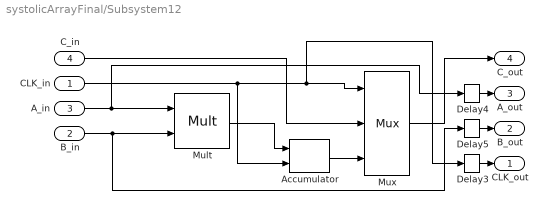
== system systolicArrayFinal/Subsystem12 ==
  CLK_in : Inport
  B_in : Inport  Port=2
  A_in : Inport  Port=3
  C_in : Inport  Port=4
  Accumulator : hdlBasic/Accumulator  operation=Add  n_bits=8  overflow=Wrap  scale=1  rst=on  hasbypass=off  en=off  latency=1  msb_inp=100  msb=100  lsb=-100  use_behavioral_HDL=on  implementation=Fabric  XmcBlockStatus=1  maskContainerNames=group3  block_type=accum  block_config=sysgen:Accum_config
  Delay3 : hdlBasic/Delay  rst=off  en=off  latency=1  reg_retiming=off  XmcBlockStatus=1  maskContainerNames=group1  block_type=delay  block_config=sysgen:Delay_config
  Delay4 : hdlBasic/Delay  rst=off  en=off  latency=1  reg_retiming=off  XmcBlockStatus=1  maskContainerNames=group1  block_type=delay  block_config=sysgen:Delay_config
  Delay5 : hdlBasic/Delay  rst=off  en=off  latency=1  reg_retiming=off  XmcBlockStatus=1  maskContainerNames=group1  block_type=delay  block_config=sysgen:Delay_config
  Mult : hdlBasic/Mult  precision=Full  arith_type="Signed  (2's comp)"  n_bits=16  bin_pt=14  quantization=Truncate  overflow=Wrap  en=off  latency=0  use_behavioral_HDL=off  opt=Speed  use_embedded=on  optimum_pipeline=off  pipeline=on  use_rpm=on  placement_style=Triangular  XmcBlockStatus=1  maskContainerNames=group1  block_type=mult  block_config=sysgen:Mult_config
  Mux : hdlBasic/Mux  inputs=2  en=off  latency=0  precision=Full  arith_type=Unsigned  n_bits=16  bin_pt=14  quantization=Truncate  overflow=Wrap  XmcBlockStatus=1  maskContainerNames=tabcontainer1  block_type=mux  block_config=sysgen:Mux_config
  CLK_out : Outport
  B_out : Outport  Port=2
  A_out : Outport  Port=3
  C_out : Outport  Port=4
  wires:
  Accumulator/1 -> Mux/3
  Mult/1 -> Accumulator/1
  Mux/1 -> C_out/1
  CLK_in/1 -> Accumulator/2, Delay3/1, Mux/1
  C_in/1 -> Mux/2
  A_in/1 -> Delay4/1, Mult/1
  B_in/1 -> Delay5/1, Mult/2
  Delay3/1 -> CLK_out/1
  Delay4/1 -> A_out/1
  Delay5/1 -> B_out/1

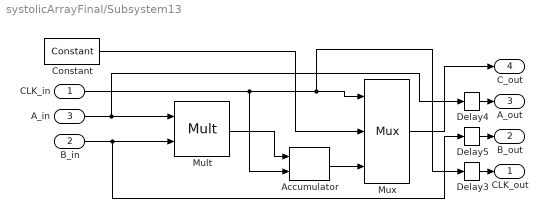
== system systolicArrayFinal/Subsystem13 ==
  CLK_in : Inport
  B_in : Inport  Port=2
  A_in : Inport  Port=3
  Accumulator : hdlBasic/Accumulator  operation=Add  n_bits=16  overflow=Wrap  scale=1  rst=on  hasbypass=off  en=off  latency=1  msb_inp=100  msb=100  lsb=-100  use_behavioral_HDL=on  implementation=Fabric  XmcBlockStatus=1  maskContainerNames=group3  block_type=accum  block_config=sysgen:Accum_config
  Constant : hdlBasic/Constant  const=0  gui_display_data_type=Fixed-point  arith_type=Signed (2's comp)  n_bits=16  bin_pt=0  preci_type=Single  exp_width=8  frac_width=24  explicit_period=off  period=1  XmcBlockStatus=1  maskContainerNames=tabcontainer1  block_type=constant  block_config=sysgen:Constant_config
  Delay3 : hdlBasic/Delay  rst=off  en=off  latency=1  reg_retiming=off  XmcBlockStatus=1  maskContainerNames=group1  block_type=delay  block_config=sysgen:Delay_config
  Delay4 : hdlBasic/Delay  rst=off  en=off  latency=1  reg_retiming=off  XmcBlockStatus=1  maskContainerNames=group1  block_type=delay  block_config=sysgen:Delay_config
  Delay5 : hdlBasic/Delay  rst=off  en=off  latency=1  reg_retiming=off  XmcBlockStatus=1  maskContainerNames=group1  block_type=delay  block_config=sysgen:Delay_config
  Mult : hdlBasic/Mult  precision=Full  arith_type="Signed  (2's comp)"  n_bits=16  bin_pt=14  quantization=Truncate  overflow=Wrap  en=off  latency=0  use_behavioral_HDL=off  opt=Speed  use_embedded=on  optimum_pipeline=off  pipeline=on  use_rpm=on  placement_style=Triangular  XmcBlockStatus=1  maskContainerNames=group1  block_type=mult  block_config=sysgen:Mult_config
  Mux : hdlBasic/Mux  inputs=2  en=off  latency=0  precision=Full  arith_type=Unsigned  n_bits=16  bin_pt=14  quantization=Truncate  overflow=Wrap  XmcBlockStatus=1  maskContainerNames=tabcontainer1  block_type=mux  block_config=sysgen:Mux_config
  CLK_out : Outport
  B_out : Outport  Port=2
  A_out : Outport  Port=3
  C_out : Outport  Port=4
  wires:
  Accumulator/1 -> Mux/3
  Mult/1 -> Accumulator/1
  Mux/1 -> C_out/1
  CLK_in/1 -> Accumulator/2, Delay3/1, Mux/1
  A_in/1 -> Delay4/1, Mult/1
  B_in/1 -> Delay5/1, Mult/2
  Delay3/1 -> CLK_out/1
  Delay4/1 -> A_out/1
  Delay5/1 -> B_out/1
  Constant/1 -> Mux/2

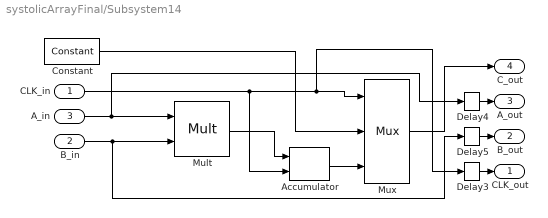
== system systolicArrayFinal/Subsystem14 ==
  CLK_in : Inport
  B_in : Inport  Port=2
  A_in : Inport  Port=3
  Accumulator : hdlBasic/Accumulator  operation=Add  n_bits=16  overflow=Wrap  scale=1  rst=on  hasbypass=off  en=off  latency=1  msb_inp=100  msb=100  lsb=-100  use_behavioral_HDL=on  implementation=Fabric  XmcBlockStatus=1  maskContainerNames=group3  block_type=accum  block_config=sysgen:Accum_config
  Constant : hdlBasic/Constant  const=0  gui_display_data_type=Fixed-point  arith_type=Signed (2's comp)  n_bits=16  bin_pt=0  preci_type=Single  exp_width=8  frac_width=24  explicit_period=off  period=1  XmcBlockStatus=1  maskContainerNames=tabcontainer1  block_type=constant  block_config=sysgen:Constant_config
  Delay3 : hdlBasic/Delay  rst=off  en=off  latency=1  reg_retiming=off  XmcBlockStatus=1  maskContainerNames=group1  block_type=delay  block_config=sysgen:Delay_config
  Delay4 : hdlBasic/Delay  rst=off  en=off  latency=1  reg_retiming=off  XmcBlockStatus=1  maskContainerNames=group1  block_type=delay  block_config=sysgen:Delay_config
  Delay5 : hdlBasic/Delay  rst=off  en=off  latency=1  reg_retiming=off  XmcBlockStatus=1  maskContainerNames=group1  block_type=delay  block_config=sysgen:Delay_config
  Mult : hdlBasic/Mult  precision=Full  arith_type="Signed  (2's comp)"  n_bits=16  bin_pt=14  quantization=Truncate  overflow=Wrap  en=off  latency=0  use_behavioral_HDL=off  opt=Speed  use_embedded=on  optimum_pipeline=off  pipeline=on  use_rpm=on  placement_style=Triangular  XmcBlockStatus=1  maskContainerNames=group1  block_type=mult  block_config=sysgen:Mult_config
  Mux : hdlBasic/Mux  inputs=2  en=off  latency=0  precision=Full  arith_type=Unsigned  n_bits=16  bin_pt=14  quantization=Truncate  overflow=Wrap  XmcBlockStatus=1  maskContainerNames=tabcontainer1  block_type=mux  block_config=sysgen:Mux_config
  CLK_out : Outport
  B_out : Outport  Port=2
  A_out : Outport  Port=3
  C_out : Outport  Port=4
  wires:
  Accumulator/1 -> Mux/3
  Mult/1 -> Accumulator/1
  Mux/1 -> C_out/1
  CLK_in/1 -> Accumulator/2, Delay3/1, Mux/1
  A_in/1 -> Delay4/1, Mult/1
  B_in/1 -> Delay5/1, Mult/2
  Delay3/1 -> CLK_out/1
  Delay4/1 -> A_out/1
  Delay5/1 -> B_out/1
  Constant/1 -> Mux/2

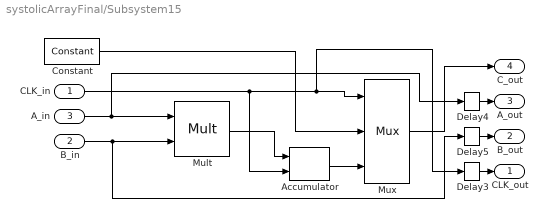
== system systolicArrayFinal/Subsystem15 ==
  CLK_in : Inport
  B_in : Inport  Port=2
  A_in : Inport  Port=3
  Accumulator : hdlBasic/Accumulator  operation=Add  n_bits=16  overflow=Wrap  scale=1  rst=on  hasbypass=off  en=off  latency=1  msb_inp=100  msb=100  lsb=-100  use_behavioral_HDL=on  implementation=Fabric  XmcBlockStatus=1  maskContainerNames=group3  block_type=accum  block_config=sysgen:Accum_config
  Constant : hdlBasic/Constant  const=0  gui_display_data_type=Fixed-point  arith_type=Signed (2's comp)  n_bits=16  bin_pt=0  preci_type=Single  exp_width=8  frac_width=24  explicit_period=off  period=1  XmcBlockStatus=1  maskContainerNames=tabcontainer1  block_type=constant  block_config=sysgen:Constant_config
  Delay3 : hdlBasic/Delay  rst=off  en=off  latency=1  reg_retiming=off  XmcBlockStatus=1  maskContainerNames=group1  block_type=delay  block_config=sysgen:Delay_config
  Delay4 : hdlBasic/Delay  rst=off  en=off  latency=1  reg_retiming=off  XmcBlockStatus=1  maskContainerNames=group1  block_type=delay  block_config=sysgen:Delay_config
  Delay5 : hdlBasic/Delay  rst=off  en=off  latency=1  reg_retiming=off  XmcBlockStatus=1  maskContainerNames=group1  block_type=delay  block_config=sysgen:Delay_config
  Mult : hdlBasic/Mult  precision=Full  arith_type="Signed  (2's comp)"  n_bits=16  bin_pt=14  quantization=Truncate  overflow=Wrap  en=off  latency=0  use_behavioral_HDL=off  opt=Speed  use_embedded=on  optimum_pipeline=off  pipeline=on  use_rpm=on  placement_style=Triangular  XmcBlockStatus=1  maskContainerNames=group1  block_type=mult  block_config=sysgen:Mult_config
  Mux : hdlBasic/Mux  inputs=2  en=off  latency=0  precision=Full  arith_type=Unsigned  n_bits=16  bin_pt=14  quantization=Truncate  overflow=Wrap  XmcBlockStatus=1  maskContainerNames=tabcontainer1  block_type=mux  block_config=sysgen:Mux_config
  CLK_out : Outport
  B_out : Outport  Port=2
  A_out : Outport  Port=3
  C_out : Outport  Port=4
  wires:
  Accumulator/1 -> Mux/3
  Mult/1 -> Accumulator/1
  Mux/1 -> C_out/1
  CLK_in/1 -> Accumulator/2, Delay3/1, Mux/1
  A_in/1 -> Delay4/1, Mult/1
  B_in/1 -> Delay5/1, Mult/2
  Delay3/1 -> CLK_out/1
  Delay4/1 -> A_out/1
  Delay5/1 -> B_out/1
  Constant/1 -> Mux/2
